simulink model "sim_new_telemetry_system"  (R2025b)
settings: Solver=VariableStepAuto  StartTime=0.0  StopTime=50.0  RelTol=1e-3
model workspace (MAT data in the model file):
  tau = Simulink.Parameter
  tau.Value = 5
  tau.Complexity = 'real'
  tau.Dimensions = [1 1]
  tau.DataType = 'auto'
undefined symbols (not defined in the file or in its folder): b_coeff, dspblkCoreblockFVToolHelper, gcbh, Rows
libraries: simulink x6, hdlsllib x3, commhdlcrc x2, dspsrcs4 x2, commseqgen3 x1, dspsigops x1
settings Model: Creator=strog  LastModifiedBy=strog

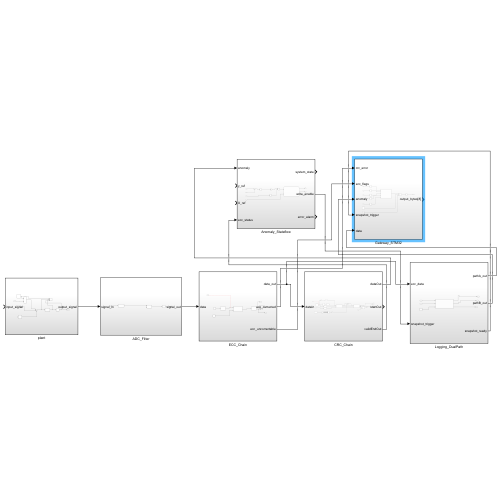
[thumbnail: Simulink's stored preview of the top-level diagram]
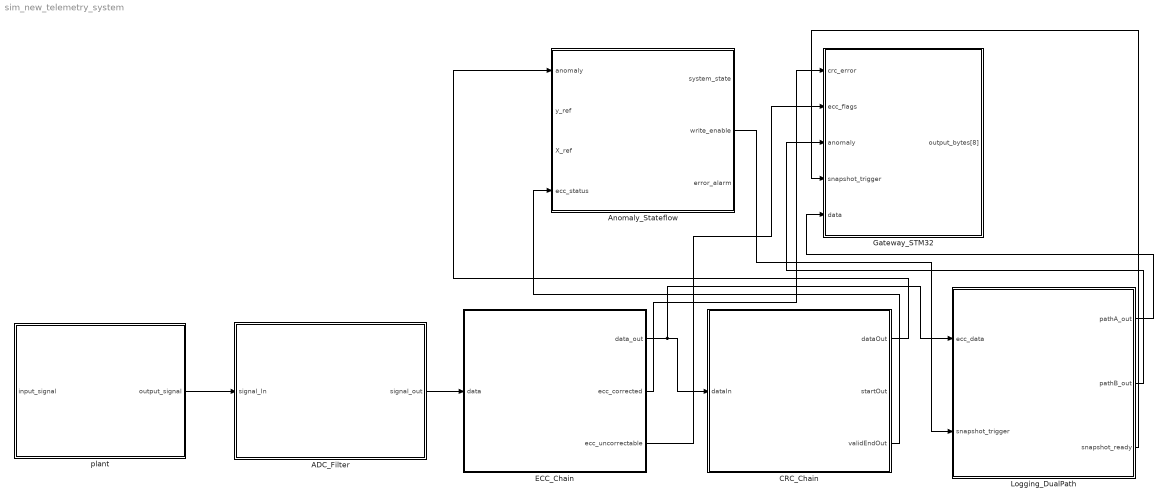
== system sim_new_telemetry_system ==
  ADC_Filter : Subsystem
  Anomaly_Stateflow : Subsystem
  CRC_Chain : Subsystem
  ECC_Chain : Subsystem
  Gateway_STM32 : Subsystem
  Logging_DualPath : Subsystem
  plant : Subsystem
  wires:
  plant/1(output_signal) -> ADC_Filter/1(signal_In)
  ADC_Filter/1(signal_out) -> ECC_Chain/1(data)
  ECC_Chain/1(data_out) -> Logging_DualPath/1(ecc_data), CRC_Chain/1(dataIn)
  CRC_Chain/1(dataOut) -> Anomaly_Stateflow/1(anomaly)
  CRC_Chain/3(validEndOut) -> Anomaly_Stateflow/4(ecc_status)
  ECC_Chain/2(ecc_corrected) -> Gateway_STM32/1(crc_error)
  Anomaly_Stateflow/2(write_enable) -> Logging_DualPath/2(snapshot_trigger)
  Logging_DualPath/1(pathA_out) -> Gateway_STM32/5(data)
  Logging_DualPath/2(pathB_out) -> Gateway_STM32/3(anomaly)
  Logging_DualPath/3(snapshot_ready) -> Gateway_STM32/4(snapshot_trigger)
  ECC_Chain/3(ecc_uncorrectable) -> Gateway_STM32/2(ecc_flags)

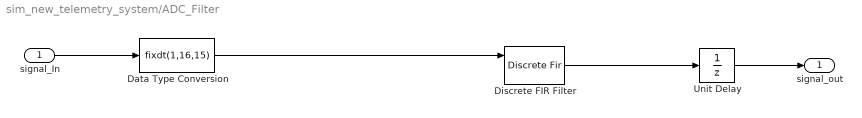
== system sim_new_telemetry_system/ADC_Filter ==
  signal_In : Inport
  Data Type Conversion : DataTypeConversion  OutDataTypeStr=fixdt(1,16,15)  RndMeth=Nearest
  Discrete FIR Filter : DiscreteFir  LoadFcn=dspblkCoreblockFVToolHelper(gcbh,'load');  Coefficients=b_coeff  ExternalReset=Level  CoefDataTypeStr=fixdt(1,16,15)  ProductDataTypeStr=fixdt(1, 32, 30)  AccumDataTypeStr=fixdt(1, 34, 30)  OutDataTypeStr=fixdt(1, 16, 15)
      settings: CopyFcn=dspblkCoreblockFVToolHelper(gcbh,'copy');  DeleteFcn=dspblkCoreblockFVToolHelper(gcbh,'close');  ModelCloseFcn=dspblkCoreblockFVToolHelper(gcbh,'close');  PreSaveFcn=dspblkCoreblockFVToolHelper(gcbh,'presave');  PostSaveFcn=dspblkCoreblockFVToolHelper(gcbh,'postsave');  CloseFcn=dspblkCoreblockFVToolHelper(gcbh,'close');  InputPortMap=u0,r6
  Unit Delay : UnitDelay  SampleTime=1e-8  HasFrameUpgradeWarning=on
  signal_out : Outport
  wires:
  Data Type Conversion/1 -> Discrete FIR Filter/1
  Discrete FIR Filter/1 -> Unit Delay/1
  signal_In/1 -> Data Type Conversion/1
  Unit Delay/1 -> signal_out/1

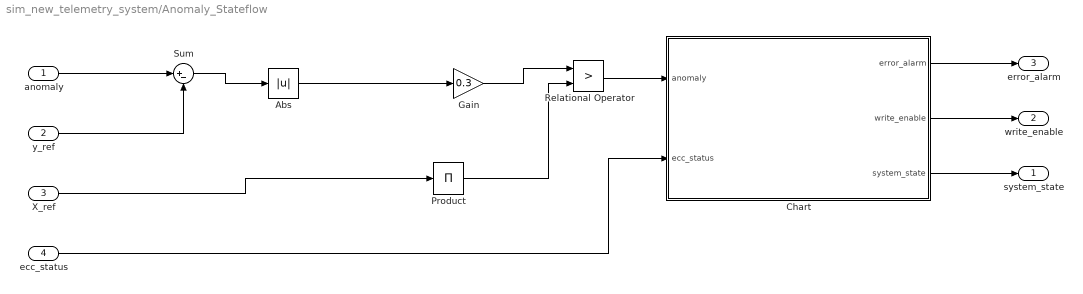
== system sim_new_telemetry_system/Anomaly_Stateflow ==
  anomaly : Inport
  y_ref : Inport  Port=2
  X_ref : Inport  Port=3
  ecc_status : Inport  Port=4
  Abs : Abs  SaturateOnIntegerOverflow=off
  Chart : Stateflow chart  TreatAsAtomicUnit=on
  Gain : Gain  Gain=0.3
  Product : Product  Inputs=1
  Relational Operator : RelationalOperator  Operator=>  OutDataTypeStr=boolean  RndMeth=Simplest  InputSameDT=off
  Sum : Sum  Inputs=|+-
  system_state : Outport
  write_enable : Outport  Port=2
  error_alarm : Outport  Port=3
  wires:
  Sum/1 -> Abs/1
  Abs/1 -> Gain/1
  Gain/1 -> Relational Operator/1
  anomaly/1 -> Sum/1
  y_ref/1 -> Sum/2
  Product/1 -> Relational Operator/2
  X_ref/1 -> Product/1
  Relational Operator/1 -> Chart/1(anomaly)
  ecc_status/1 -> Chart/2(ecc_status)
  Chart/3(system_state) -> system_state/1
  Chart/2(write_enable) -> write_enable/1
  Chart/1(error_alarm) -> error_alarm/1

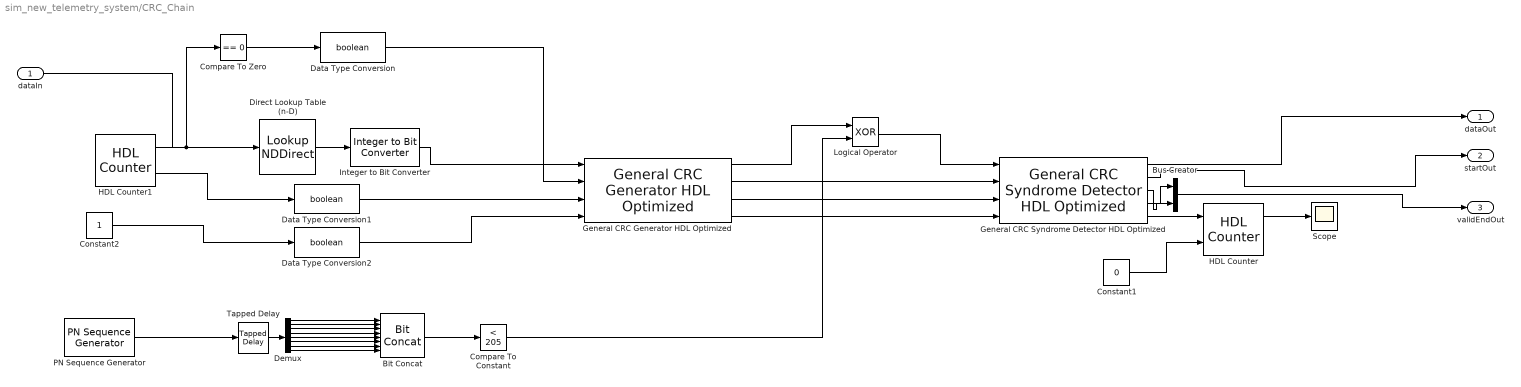
== system sim_new_telemetry_system/CRC_Chain ==
  dataIn : Inport
  Bit Concat : hdlsllib/Logic and Bit Operations/Bit Concat  numInputs=8
  Bus Creator : BusCreator  Inputs=2
  Compare To Constant : simulink/Logic and Bit Operations/Compare To Constant  relop=<  const=205  OutDataTypeStr=boolean
  Compare To Zero : simulink/Logic and Bit Operations/Compare To Zero  relop===  OutDataTypeStr=boolean
  Constant1 : Constant  Value=0  OutDataTypeStr=boolean
  Constant2 : Constant  OutDataTypeStr=boolean
  Data Type Conversion : DataTypeConversion  OutDataTypeStr=boolean  SaturateOnIntegerOverflow=off  RndMeth=Floor
  Data Type Conversion1 : DataTypeConversion  OutDataTypeStr=boolean  SaturateOnIntegerOverflow=off  RndMeth=Floor
  Data Type Conversion2 : DataTypeConversion  OutDataTypeStr=boolean  SaturateOnIntegerOverflow=off  RndMeth=Floor
  Demux : Demux  Outputs=8
  Direct Lookup Table (n-D) : LookupNDDirect  NumberOfTableDimensions=1  Table=[72, 101, 108, 108, 111]  TableDataTypeStr=uint8
  General CRC Generator HDL Optimized : commhdlcrc/General CRC Generator HDL Optimized  Polynomial=polyCoeffs  InitialState=1  DirectMethod=on  ReflectInput=on  ReflectCRCChecksum=on  FinalXORValue=ones(1, 32)  SimulateUsing=Code generation
  General CRC Syndrome Detector HDL Optimized : commhdlcrc/General CRC Syndrome Detector HDL Optimized  Polynomial=polyCoeffs  InitialState=1  DirectMethod=on  ReflectInput=on  ReflectCRCChecksum=on  FinalXORValue=ones(1, 32)  SimulateUsing=Code generation
  HDL Counter : hdlsllib/Sources/HDL Counter  CountType=Count limited  CountInit=0  CountStep=1  CountMax=25  CountFromType=Initial value  CountFrom=0  CountResetPort=on  CountLoadPort=off  CountEnbPort=on  CountDirPort=off  CountHitOutputPort=on  CountDataType=Unsigned  CountWordLen=8  CountFracLen=0  CountSampTime=uint8(1)
  HDL Counter1 : hdlsllib/Sources/HDL Counter  CountType=Count limited  CountInit=0  CountStep=1  CountMax=4  CountFromType=Initial value  CountFrom=0  CountResetPort=off  CountLoadPort=off  CountEnbPort=off  CountDirPort=off  CountHitOutputPort=on  CountDataType=Unsigned  CountWordLen=8  CountFracLen=0  CountSampTime=1
  Integer to Bit Converter : simulink/Logic and Bit Operations/Integer to Bit Converter  nbits=8  signedInputValues=Unsigned  bitOrder=MSB first  outDtype=boolean
      settings: LibrarySourceBlock=|
      | commutil2/Integer to Bit
      | Converter
  Logical Operator : Logic  Operator=XOR  AllPortsSameDT=off  OutDataTypeStr=boolean
  PN Sequence Generator : commseqgen3/PN Sequence Generator  poly='z^6 + z + 1'  ini_sta=[0 0 0 0 0 1]  outBitMaskSource=Dialog parameter  shift=0  outVarSiz=off  maxOutSizeMode=Dialog parameter  maxOutSize=[10 1]  Ts=1  sampPerFrame=1  reset=off  bitPackedOutputs=off  outDataType=boolean  numPackedBits=8  bitPackDataSigned=off  bitPackedOutDType=double
      settings: LibrarySourceBlock=|
      | commhdlsource/PN Sequence
      | Generator
  Scope : Scope
      settings: ActiveDisplayYMinimum=-1  ActiveDisplayYMaximum=1  DataLoggingSaveFormat=Array
  Tapped Delay : simulink/Discrete/Tapped Delay  vinit=0.0  samptime=-1  NumDelays=8  DelayOrder=Oldest  includeCurrent=off
  dataOut : Outport
  startOut : Outport  Port=2
  validEndOut : Outport  Port=3
  wires:
  Data Type Conversion/1 -> General CRC Generator HDL Optimized/2
  Data Type Conversion1/1 -> General CRC Generator HDL Optimized/3
  Integer to Bit Converter/1 -> General CRC Generator HDL Optimized/1
  Logical Operator/1 -> General CRC Syndrome Detector HDL Optimized/1
  General CRC Syndrome Detector HDL Optimized/1 -> dataOut/1
  HDL Counter1/2 -> Data Type Conversion1/1
  Demux/1 -> Bit Concat/1
  Demux/7 -> Bit Concat/7
  Demux/2 -> Bit Concat/2
  General CRC Generator HDL Optimized/4 -> General CRC Syndrome Detector HDL Optimized/4
  HDL Counter/1 -> Scope/1
  Bus Creator/1 -> validEndOut/1
  Demux/4 -> Bit Concat/4
  Demux/8 -> Bit Concat/8
  HDL Counter1/1 -> Compare To Zero/1, Direct Lookup Table (n-D)/1
  Constant1/1 -> HDL Counter/2
  Bit Concat/1 -> Compare To Constant/1
  Data Type Conversion2/1 -> General CRC Generator HDL Optimized/4
  Direct Lookup Table (n-D)/1 -> Integer to Bit Converter/1
  General CRC Generator HDL Optimized/1 -> Logical Operator/1
  Demux/5 -> Bit Concat/5
  Demux/6 -> Bit Concat/6
  General CRC Syndrome Detector HDL Optimized/4 -> Bus Creator/1
  General CRC Syndrome Detector HDL Optimized/3 -> Bus Creator/2
  General CRC Syndrome Detector HDL Optimized/2 -> startOut/1
  Constant2/1 -> Data Type Conversion2/1
  PN Sequence Generator/1 -> Tapped Delay/1
  Demux/3 -> Bit Concat/3
  Tapped Delay/1 -> Demux/1
  General CRC Generator HDL Optimized/3 -> General CRC Syndrome Detector HDL Optimized/3
  Compare To Constant/1 -> Logical Operator/2
  Compare To Zero/1 -> Data Type Conversion/1
  General CRC Syndrome Detector HDL Optimized/5 -> HDL Counter/1
  General CRC Generator HDL Optimized/2 -> General CRC Syndrome Detector HDL Optimized/2
  dataIn/1 -> ?

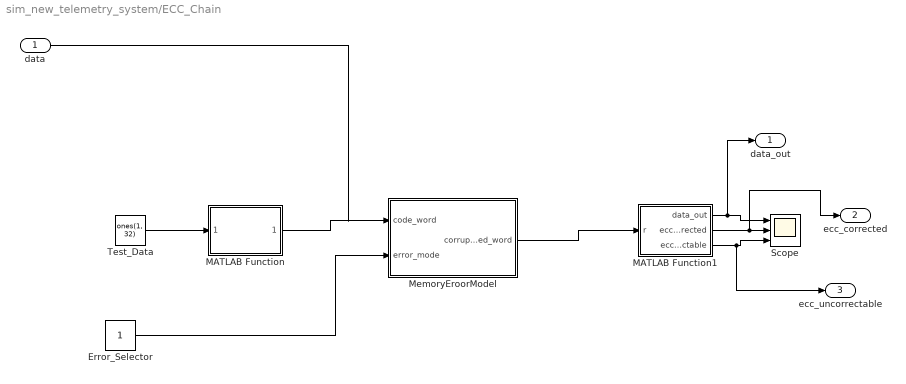
== system sim_new_telemetry_system/ECC_Chain ==
  data : Inport
  Error_Selector : Constant  OutDataTypeStr=boolean
  MATLAB Function : MATLAB Function  TreatAsAtomicUnit=on
  MATLAB Function1 : MATLAB Function  TreatAsAtomicUnit=on
  MemoryEroorModel : Subsystem
  Scope : Scope  NumInputPorts=3
      settings: DataLoggingSaveFormat=Array
  Test_Data : Constant  Value=ones(1, 32)  OutDataTypeStr=boolean
  data_out : Outport
  ecc_corrected : Outport  Port=2
  ecc_uncorrectable : Outport  Port=3
  wires:
  Test_Data/1 -> MATLAB Function/1(data_in)
  MemoryEroorModel/1(corrupted_word) -> MATLAB Function1/1(r)
  MATLAB Function/1(code_word) -> MemoryEroorModel/1(code_word)
  Error_Selector/1 -> MemoryEroorModel/2(error_mode)
  MATLAB Function1/2(ecc_corrected) -> ecc_corrected/1, Scope/2
  MATLAB Function1/1(data_out) -> data_out/1, Scope/1
  MATLAB Function1/3(ecc_uncorrectable) -> ecc_uncorrectable/1, Scope/3
  data/1 -> ?

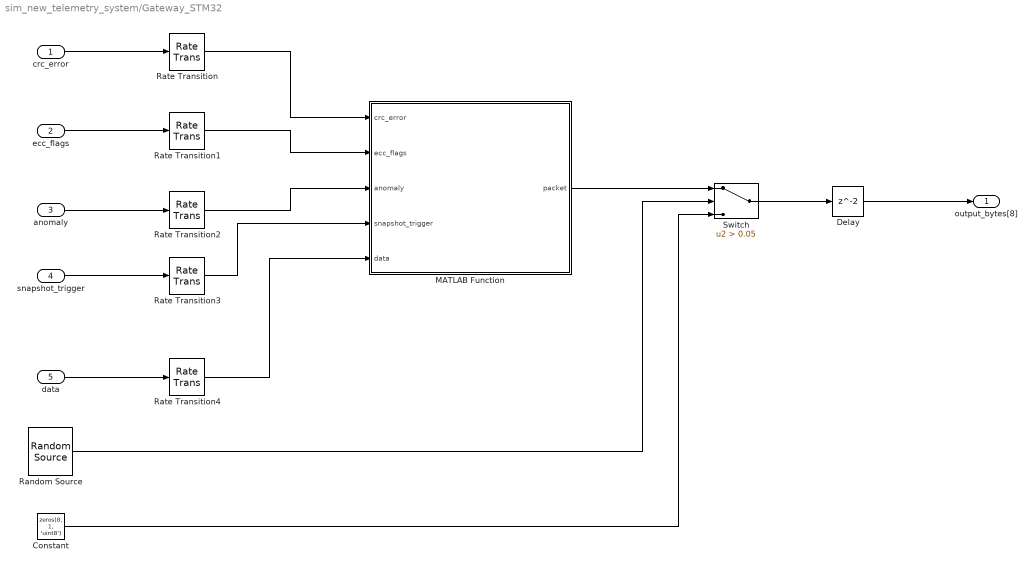
== system sim_new_telemetry_system/Gateway_STM32 ==
  crc_error : Inport  OutDataTypeStr=boolean
  ecc_flags : Inport  Port=2  OutDataTypeStr=uint8
  anomaly : Inport  Port=3  OutDataTypeStr=boolean
  snapshot_trigger : Inport  Port=4  OutDataTypeStr=boolean
  data : Inport  Port=5  OutDataTypeStr=double
  Constant : Constant  Value=zeros(8, 1, 'uint8')
  Delay : Delay
  MATLAB Function : MATLAB Function  TreatAsAtomicUnit=on
  Random Source : dspsrcs4/Random Source  SrcType=Uniform  MinVal=0  MaxVal=1  MeanVal=0  VarVal=1  RepMode=Specify seed  rawSeed=1  IsInherit=off  SampTime=0.01  SampFrame=1  OutComplex=Real  DataType=double  SimulateUsing=Interpreted execution
  Rate Transition{,1..4} (5 alike) : RateTransition  OutPortSampleTime=0.01
  Switch : Switch  Criteria=u2 > Threshold  Threshold=0.05  SaturateOnIntegerOverflow=off  InputSameDT=off
  output_bytes[8] : Outport
  wires:
  MATLAB Function/1(packet) -> Switch/1
  data/1 -> Rate Transition4/1
  Delay/1 -> output_bytes[8]/1
  Rate Transition/1 -> MATLAB Function/1(crc_error)
  Rate Transition1/1 -> MATLAB Function/2(ecc_flags)
  ecc_flags/1 -> Rate Transition1/1
  Rate Transition4/1 -> MATLAB Function/5(data)
  crc_error/1 -> Rate Transition/1
  Rate Transition2/1 -> MATLAB Function/3(anomaly)
  Switch/1 -> Delay/1
  Random Source/1 -> Switch/2
  Rate Transition3/1 -> MATLAB Function/4(snapshot_trigger)
  anomaly/1 -> Rate Transition2/1
  Constant/1 -> Switch/3
  snapshot_trigger/1 -> Rate Transition3/1

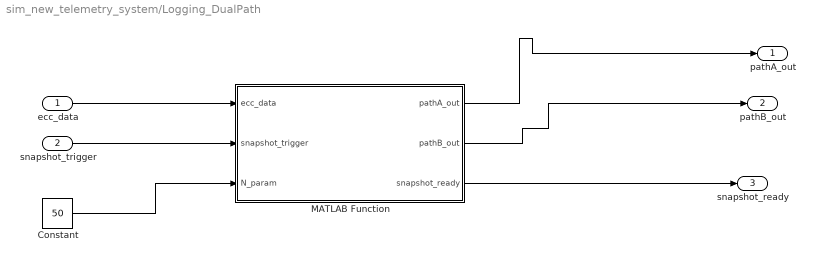
== system sim_new_telemetry_system/Logging_DualPath ==
  ecc_data : Inport
  snapshot_trigger : Inport  Port=2
  Constant : Constant  Value=50
  MATLAB Function : MATLAB Function  TreatAsAtomicUnit=on
  pathA_out : Outport  PortDimensions=1
  pathB_out : Outport  Port=2  PortDimensions=100
  snapshot_ready : Outport  Port=3
  wires:
  MATLAB Function/1(pathA_out) -> pathA_out/1
  snapshot_trigger/1 -> MATLAB Function/2(snapshot_trigger)
  Constant/1 -> MATLAB Function/3(N_param)
  ecc_data/1 -> MATLAB Function/1(ecc_data)
  MATLAB Function/2(pathB_out) -> pathB_out/1
  MATLAB Function/3(snapshot_ready) -> snapshot_ready/1

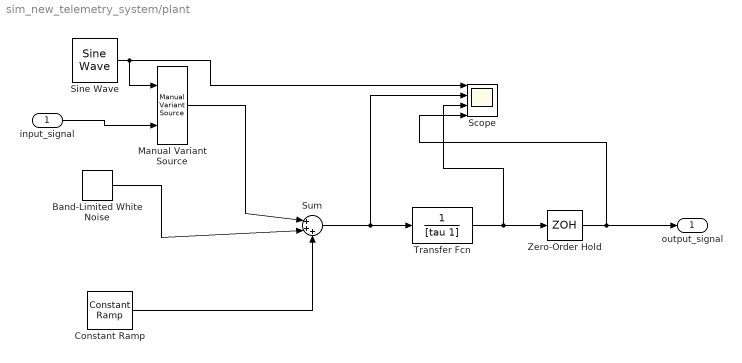
== system sim_new_telemetry_system/plant ==
  input_signal : Inport
  Band-Limited White Noise : simulink/Sources/Band-Limited White Noise  Cov=[0.1]  Ts=0.1  seed=[23341]
  Constant Ramp : dspsigops/Constant Ramp  L=Rows  dim=1  Slope=0.001  dataType=Same as input  isSigned=on  wordLen=16  udDataType=sfix(16)  fracBitsMode=Best precision  numFracBits=15  Offset=0
  Manual Variant Source : simulink/Signal Routing/Manual Variant Source  NumChoices=2  LabelModeActiveChoice=V_1
  Scope : Scope  NumInputPorts=4
      settings: DataLoggingVariableName=ScopeData2  DataLoggingSaveFormat=Array
  Sine Wave : dspsrcs4/Sine Wave  Amplitude=1  Frequency=1  Phase=0  SampleMode=Discrete  OutComplex=Real  CompMethod=Trigonometric fcn  TableSize=Speed  SampleTime=1/1000  SamplesPerFrame=1  ResetState=Restart at time zero  OutputFrames=off  dataType=double  wordLen=16  udDataType=sfix(16)  fracBitsMode=Best precision  numFracBits=15  OutDataTypeStr=double  LastOutDataTypeStr=double
  Sum : Sum  Inputs=|+++
  Transfer Fcn : TransferFcn  Denominator=[tau 1]
  Zero-Order Hold : ZeroOrderHold  SampleTime=0.01
  output_signal : Outport
  wires:
  Sine Wave/1 -> Manual Variant Source/1, Scope/1
  Band-Limited White Noise/1 -> Sum/2
  Constant Ramp/1 -> Sum/3
  Sum/1 -> Scope/2, Transfer Fcn/1
  Transfer Fcn/1 -> Scope/3, Zero-Order Hold/1
  Zero-Order Hold/1 -> Scope/4, output_signal/1
  input_signal/1 -> Manual Variant Source/2
  Manual Variant Source/1 -> Sum/1

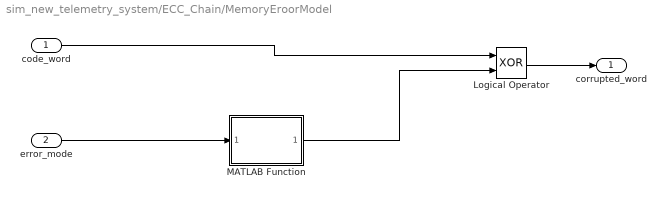
== system sim_new_telemetry_system/ECC_Chain/MemoryEroorModel ==
  code_word : Inport
  error_mode : Inport  Port=2
  Logical Operator : Logic  Operator=XOR  AllPortsSameDT=off  OutDataTypeStr=boolean
  MATLAB Function : MATLAB Function  TreatAsAtomicUnit=on
  corrupted_word : Outport
  wires:
  code_word/1 -> Logical Operator/1
  error_mode/1 -> MATLAB Function/1(error_mode)
  MATLAB Function/1(error_mask) -> Logical Operator/2
  Logical Operator/1 -> corrupted_word/1

== matlab function sim_new_telemetry_system/ECC_Chain/MATLAB Function1 ==
  data: r input; data_out output; ecc_corrected output; ecc_uncorrectable output
function [data_out, ecc_corrected, ecc_uncorrectable] = fcn(r)
    % r: принятое из памяти 39-битное слово
    
    % Инициализация флагов
    ecc_corrected = 0;
    ecc_uncorrectable = 0;
    
    % 1. Вычисляем синдром Хэмминга (6 бит)
    s = zeros(1, 6);
    s(1) = mod(sum(r([1, 3, 5, 7, 9, 11, 13, 15, 17, 19, 21, 23, 25, 27, 29, 31, 33, 35, 37])), 2);
    s(2) = mod(sum(r([2, 3, 6, 7, 10, 11, 14, 15, 18, 19, 22, 23, 26, 27, 30, 31, 34, 35, 38])), 2);
    s(3) = mod(sum(r([4, 5, 6, 7, 12, 13, 14, 15, 20, 21, 22, 23, 28, 29, 30, 31, 36, 37, 38])), 2);
    s(4) = mod(sum(r([8:15, 24:31, 38])), 2);
    s(5) = mod(sum(r([16:31])), 2);
    s(6) = mod(sum(r([32:38])), 2);
    
    % Преобразуем синдром в десятичное число (индекс ошибочного бита)
    syndrome_val = s(1)*1 + s(2)*2 + s(3)*4 + s(4)*8 + s(5)*16 + s(6)*32;
    
    % 2. Вычисляем общий паритет принятого слова
    overall_parity = mod(sum(r), 2); % Если ошибок нет, общий паритет должен быть равен 0
    
    % 3. Логика SECDED декодирования
    if syndrome_val == 0
        if overall_parity == 0
            % Ошибок нет
        else
            % Ошибка в самом бите общего паритета (39)
            r(39) = mod(r(39) + 1, 2);
            ecc_corrected = 1;
        end
    else
        if overall_parity == 1
            % Одиночная ошибка (SEC) — исправляем её
            if syndrome_val <= 39
                r(syndrome_val) = mod(r(syndrome_val) + 1, 2);
                ecc_corrected = 1;
            end
        else
            % Двойная ошибка (DED) — обнаружена, но неисправима
            ecc_uncorrectable = 1;
        end
    end
    
    % Извлекаем чистые 32 бита данных из исправленного слова
    data_pos =;
    data_out = zeros(1, 32);
    for i = 1:32
        data_out(i) = r(data_pos(i));
    end
end

== matlab function sim_new_telemetry_system/ECC_Chain/MATLAB Function ==
  data: data_in input; code_word output
function code_word = fcn(data_in)
    % data_in: вектор из 32 элементов (uint8 или логический), содержащий биты данных
    % code_word: выходной вектор из 39 бит
    
    % Инициализируем кодовое слово нулями
    c = zeros(1, 39);
    
    % Размещаем 32 бита информационных данных на позиции, не являющиеся степенями двойки
    % Позиции контрольных бит: 1, 2, 4, 8, 16, 32
    % Позиция 39 — общий бит четности (для превращения SEC в SECDED)
    
    data_pos =;
    
    for i = 1:32
        c(data_pos(i)) = data_in(i);
    end
    
    % Вычисляем контрольные биты Хэмминга (XOR по соответствующим позициям)
    c(1)  = mod(sum(c([3, 5, 7, 9, 11, 13, 15, 17, 19, 21, 23, 25, 27, 29, 31, 33, 35, 37])), 2);
    c(2)  = mod(sum(c([3, 6, 7, 10, 11, 14, 15, 18, 19, 22, 23, 26, 27, 30, 31, 34, 35, 38])), 2);
    c(4)  = mod(sum(c([5, 6, 7, 12, 13, 14, 15, 20, 21, 22, 23, 28, 29, 30, 31, 36, 37, 38])), 2);
    c(8)  = mod(sum(c([9:15, 24:31, 38])), 2); % для сокращенного кода проверяем доступные диапазоны
    c(16) = mod(sum(c([17:31])), 2);
    c(32) = mod(sum(c([33:38])), 2);
    
    % 39-й бит: Общий паритет (SECDED) — XOR всех предыдущих 38 бит
    c(39) = mod(sum(c(1:38)), 2);
    
    code_word = c;
end

== matlab function sim_new_telemetry_system/ECC_Chain/MemoryEroorModel/MATLAB Function ==
  data: error_mode input; error_mask output
function error_mask = fcn(error_mode)
    % error_mode: 0, 1 или 2
    % error_mask: вектор из 39 бит (0 или 1)
    
    error_mask = zeros(1, 39);
    
    if error_mode == 1
        % Вносим ровно 1 ошибку в фиксированную (например, 5-ю) позицию
        error_mask(5) = 1; 
    elseif error_mode == 2
        % Вносим ровно 2 ошибки (например, в 5-ю и 12-ю позиции)
        error_mask(5) = 1;
        error_mask(12) = 1;
    end
end

== stateflow chart sim_new_telemetry_system/Anomaly_Stateflow/Chart ==
  state Error
    entry:
    write_enable = false;
    error_alarm = true;
    system_state = 5;
  state Normal
    entry:
    write_enable = false;
    error_alarm = false;
    system_state = 1;
  state Snapshot
    entry:
    write_enable = true;
    system_state = 3;
  state RetryECC
    entry:
    write_enable = false;
    system_state = 4;
  state Alarm
    entry:
    anomaly_counter = 0;
    during:
    if anomaly
    anomaly_counter = anomaly_counter + 1;
    else
    anomaly_counter = 0;
    end
    system_state=2;
  (default) -> Normal
  RetryECC -> Error [order 2] : [ecc_status==2]
  RetryECC -> Normal [order 3] : [ecc_status == 0 | (ecc_status == 1 & ~anomaly)]
  Alarm -> Normal [order 2] : [~anomaly]
  Normal -> Alarm : [anomaly]
  Snapshot -> RetryECC
  Alarm -> Snapshot [order 1] : [anomaly_counter>=3]
  RetryECC -> Alarm [order 1] : [ecc_status ==1 & anomaly]
  data: anomaly input; ecc_status input; error_alarm output; write_enable output; anomaly_counter local; system_state output

== matlab function sim_new_telemetry_system/Logging_DualPath/MATLAB Function ==
  data: ecc_data input; pathA_out output size=1; snapshot_trigger input; N_param input; pathB_out output size=100; snapshot_ready output
function [pathA_out, pathB_out, snapshot_ready] = fcn(ecc_data, snapshot_trigger, N_param)
% #codegen

length_N = 50; 
total_window = length_N * 2;

persistent ring_buffer;    
persistent sample_counter; 
persistent hold_counter;   
persistent is_recording;   
persistent final_snapshot; 

if isempty(ring_buffer)
    ring_buffer = zeros(total_window, 1); % Вектор-столбец
    sample_counter = 0;
    hold_counter = 0;
    is_recording = false;
    final_snapshot = zeros(total_window, 1);
end

%% ==================== PATH A ====================
sample_counter = sample_counter + 1;
if sample_counter >= 1000
    pathA_out = ecc_data;
    sample_counter = 0;
else
    pathA_out = 0.0; 
end

%% ==================== PATH B ====================
% Сдвиг через точку с запятой для вертикального вектора
ring_buffer = [ring_buffer(2:end); ecc_data];

snapshot_ready = false;

if snapshot_trigger && ~is_recording
    is_recording = true;
    hold_counter = 0;
end

if is_recording
    hold_counter = hold_counter + 1;
    if hold_counter >= length_N
        final_snapshot = ring_buffer; 
        is_recording = false;         
        hold_counter = 0;
        snapshot_ready = true;        
    end
end

pathB_out = final_snapshot;

== matlab function sim_new_telemetry_system/Gateway_STM32/MATLAB Function ==
  data: crc_error input; packet output; ecc_flags input; anomaly input; snapshot_trigger input; data input
function packet = pack_gateway_data(crc_error, ecc_flags, anomaly, snapshot_trigger, data)
%#codegen

% Явно создаем выходной массив байт фиксированного размера
packet = zeros(8, 1, 'uint8');

% Побайтовая упаковка (кодирование) данных
packet(1) = uint8(crc_error);
packet(2) = uint8(ecc_flags);
packet(3) = uint8(anomaly);
packet(4) = uint8(snapshot_trigger);

% Преобразование single (float) в 4 байта uint8 с помощью typecast
data_bytes = typecast(single(data), 'uint8');
packet(5) = data_bytes(1);
packet(6) = data_bytes(2);
packet(7) = data_bytes(3);
packet(8) = data_bytes(4);
end
